simulink model "Bands8"  (R2018a)
settings: Solver=VariableStepAuto  StartTime=0.0  StopTime=0.007  RelTol=1e-3
undefined symbols (not defined in the file): fdesignblkfcn, G1, G2, G3, G4, G5, G6, G7, G8, gcbh, get, T
libraries: dspsrcs4 x1, dspxfrm3 x1, dspobslib x1
(part 1 of 3)
settings Model: Creator=Daniel  LastModifiedBy=Daniel

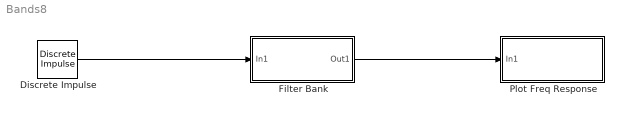
== system Bands8 ==
  Discrete Impulse : dspsrcs4/Discrete  Impulse  Delay=0  SampleTime=T  FrameSample=128  OutputFrames=off  dataType=double  isSigned=on  wordLen=16  udDataType=sfix(16)  fracBitsMode=Best precision  numFracBits=15  OutDataTypeStr=double  LastOutDataTypeStr=double
  "Filter Bank " : Subsystem
  Plot Freq Response : Subsystem
  wires:
  "Filter Bank "/1(Out1) -> Plot Freq Response/1(In1)
  Discrete Impulse/1 -> "Filter Bank "/1(In1)

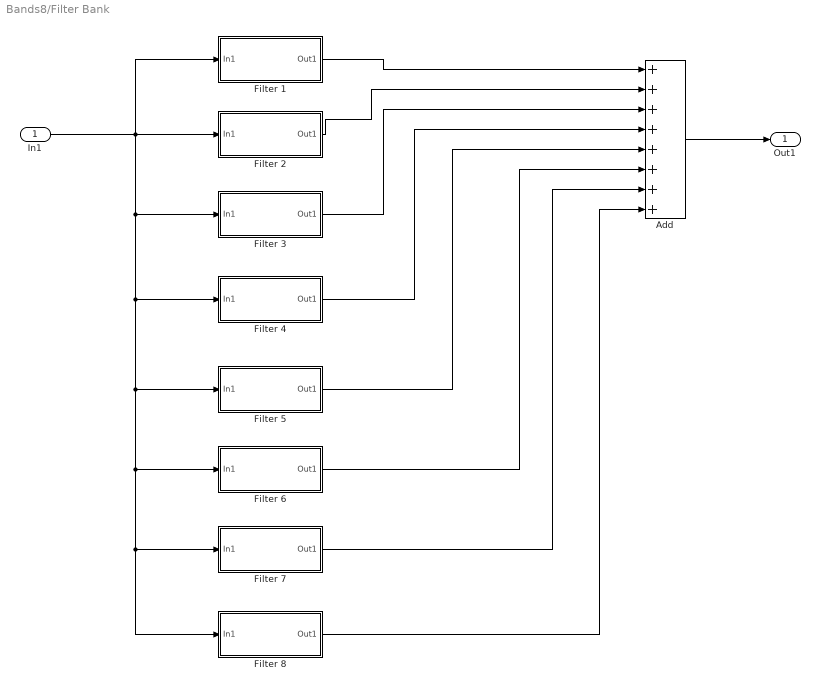
== system Bands8/Filter Bank  ==
  In1 : Inport
  Add : Sum  Inputs=++++++++
  Filter 1 : Subsystem
  Filter 2 : Subsystem
  Filter 3 : Subsystem
  Filter 4 : Subsystem
  Filter 5 : Subsystem
  Filter 6 : Subsystem
  Filter 7 : Subsystem
  Filter 8 : Subsystem
  Out1 : Outport
  wires:
  In1/1 -> Filter 3/1(In1), Filter 6/1(In1), Filter 8/1(In1), Filter 7/1(In1), Filter 5/1(In1), Filter 4/1(In1), Filter 1/1(In1), Filter 2/1(In1)
  Add/1 -> Out1/1
  Filter 1/1(Out1) -> Add/1
  Filter 2/1(Out1) -> Add/2
  Filter 3/1(Out1) -> Add/3
  Filter 4/1(Out1) -> Add/4
  Filter 5/1(Out1) -> Add/5
  Filter 6/1(Out1) -> Add/6
  Filter 7/1(Out1) -> Add/7
  Filter 8/1(Out1) -> Add/8

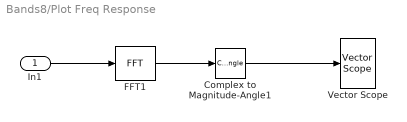
== system Bands8/Plot Freq Response ==
  In1 : Inport
  Complex to Magnitude-Angle1 : ComplexToMagnitudeAngle  Output=Magnitude
  FFT1 : dspxfrm3/FFT  FFTImplementation=Auto  CompMethod=Table lookup  TableOpt=NEW  TableOptActive=Speed  BitRevOrder=off  Normalize=off  InheritFFTLength=on  FFTLength=64  WrapInput=on  roundingMode=Floor  overflowMode=off  firstCoeffDataTypeStr=Inherit: Same word length as input  firstCoeffLastDataTypeStr=Inherit: Same word length as input  outputMin=[]  outputMax=[]
  Vector Scope : dspobslib/Vector Scope  ScopeProperties=off  Domain=Frequency  HorizSpan=1  DisplayProperties=off  AxisGrid=on  Memory=off  FrameNumber=off  AxisLegend=off  AxisZoom=off  OpenScopeAtSimStart=on  OpenScopeImmediately=off  FigPos=get(0,'defaultfigureposition')  AxisProperties=on  XUnits=Hertz  XRange=[0...Fs/2]  InheritXIncr=on  XIncr=1  XLabel=Samples  XLimit=Auto  XMin=0  XMax=1  XStart=0  YUnits=dB  YLabel=|Magnitude (dB)|  LineProperties=off  XAxisParamsVer=6.9
      settings: SourceProductName=DSP System Toolbox  SourceProductBaseCode=DS  YMin=0.0723692553519949  YMax=69.3188381671759
  wires:
  In1/1 -> FFT1/1
  FFT1/1 -> Complex to Magnitude-Angle1/1
  Complex to Magnitude-Angle1/1 -> Vector Scope/1

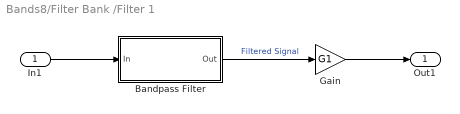
== system Bands8/Filter Bank /Filter 1 ==
  In1 : Inport
  Bandpass Filter : Subsystem  DialogController=fdesignblkfcn  InitFcn=fdesignblkfcn(gcbh, {'InitFcn'});  mask(Bandpass Filter){}
      mask help: Design a bandpass filter
      settings: CopyFcn=fdesignblkfcn(gcbh, {'CopyFcn'});
      mask Help: helpview(mapfilelocation('dsp'), 'dspbandpassfilter');
      mask Display: disp('Bandpass');
  Gain : Gain  Gain=G1
  Out1 : Outport
  wires:
  Bandpass Filter/1(Out) -> Gain/1  "Filtered Signal"
  In1/1 -> Bandpass Filter/1(In)
  Gain/1 -> Out1/1

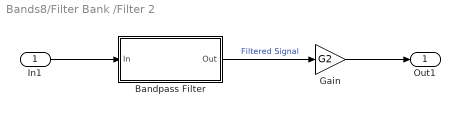
== system Bands8/Filter Bank /Filter 2 ==
  In1 : Inport
  Bandpass Filter : Subsystem  DialogController=fdesignblkfcn  InitFcn=fdesignblkfcn(gcbh, {'InitFcn'});  mask(Bandpass Filter){}
      mask help: Design a bandpass filter
      settings: CopyFcn=fdesignblkfcn(gcbh, {'CopyFcn'});
      mask Help: helpview(mapfilelocation('dsp'), 'dspbandpassfilter');
      mask Display: disp('Bandpass');
  Gain : Gain  Gain=G2
  Out1 : Outport
  wires:
  Bandpass Filter/1(Out) -> Gain/1  "Filtered Signal"
  In1/1 -> Bandpass Filter/1(In)
  Gain/1 -> Out1/1

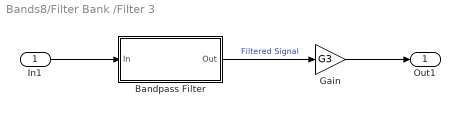
== system Bands8/Filter Bank /Filter 3 ==
  In1 : Inport
  Bandpass Filter : Subsystem  DialogController=fdesignblkfcn  InitFcn=fdesignblkfcn(gcbh, {'InitFcn'});  mask(Bandpass Filter){}
      mask help: Design a bandpass filter
      settings: CopyFcn=fdesignblkfcn(gcbh, {'CopyFcn'});
      mask Help: helpview(mapfilelocation('dsp'), 'dspbandpassfilter');
      mask Display: disp('Bandpass');
  Gain : Gain  Gain=G3
  Out1 : Outport
  wires:
  Bandpass Filter/1(Out) -> Gain/1  "Filtered Signal"
  In1/1 -> Bandpass Filter/1(In)
  Gain/1 -> Out1/1

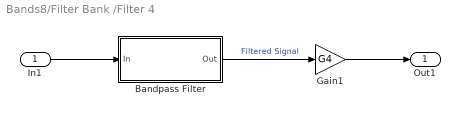
== system Bands8/Filter Bank /Filter 4 ==
  In1 : Inport
  Bandpass Filter : Subsystem  DialogController=fdesignblkfcn  InitFcn=fdesignblkfcn(gcbh, {'InitFcn'});  mask(Bandpass Filter){}
      mask help: Design a bandpass filter
      settings: CopyFcn=fdesignblkfcn(gcbh, {'CopyFcn'});
      mask Help: helpview(mapfilelocation('dsp'), 'dspbandpassfilter');
      mask Display: disp('Bandpass');
  Gain1 : Gain  Gain=G4
  Out1 : Outport
  wires:
  Bandpass Filter/1(Out) -> Gain1/1  "Filtered Signal"
  In1/1 -> Bandpass Filter/1(In)
  Gain1/1 -> Out1/1

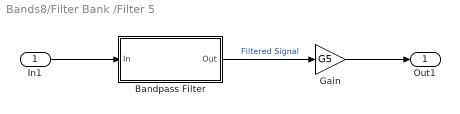
== system Bands8/Filter Bank /Filter 5 ==
  In1 : Inport
  Bandpass Filter : Subsystem  DialogController=fdesignblkfcn  InitFcn=fdesignblkfcn(gcbh, {'InitFcn'});  mask(Bandpass Filter){}
      mask help: Design a bandpass filter
      settings: CopyFcn=fdesignblkfcn(gcbh, {'CopyFcn'});
      mask Help: helpview(mapfilelocation('dsp'), 'dspbandpassfilter');
      mask Display: disp('Bandpass');
  Gain : Gain  Gain=G5
  Out1 : Outport
  wires:
  Bandpass Filter/1(Out) -> Gain/1  "Filtered Signal"
  In1/1 -> Bandpass Filter/1(In)
  Gain/1 -> Out1/1

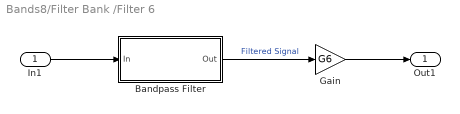
== system Bands8/Filter Bank /Filter 6 ==
  In1 : Inport
  Bandpass Filter : Subsystem  DialogController=fdesignblkfcn  InitFcn=fdesignblkfcn(gcbh, {'InitFcn'});  mask(Bandpass Filter){}
      mask help: Design a bandpass filter
      settings: CopyFcn=fdesignblkfcn(gcbh, {'CopyFcn'});
      mask Help: helpview(mapfilelocation('dsp'), 'dspbandpassfilter');
      mask Display: disp('Bandpass');
  Gain : Gain  Gain=G6
  Out1 : Outport
  wires:
  Bandpass Filter/1(Out) -> Gain/1  "Filtered Signal"
  In1/1 -> Bandpass Filter/1(In)
  Gain/1 -> Out1/1

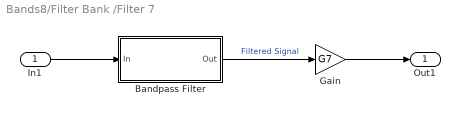
== system Bands8/Filter Bank /Filter 7 ==
  In1 : Inport
  Bandpass Filter : Subsystem  DialogController=fdesignblkfcn  InitFcn=fdesignblkfcn(gcbh, {'InitFcn'});  mask(Bandpass Filter){}
      mask help: Design a bandpass filter
      settings: CopyFcn=fdesignblkfcn(gcbh, {'CopyFcn'});
      mask Help: helpview(mapfilelocation('dsp'), 'dspbandpassfilter');
      mask Display: disp('Bandpass');
  Gain : Gain  Gain=G7
  Out1 : Outport
  wires:
  Bandpass Filter/1(Out) -> Gain/1  "Filtered Signal"
  In1/1 -> Bandpass Filter/1(In)
  Gain/1 -> Out1/1

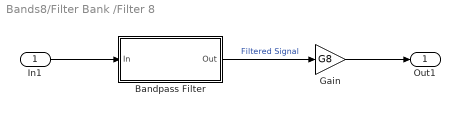
== system Bands8/Filter Bank /Filter 8 ==
  In1 : Inport
  Bandpass Filter : Subsystem  DialogController=fdesignblkfcn  InitFcn=fdesignblkfcn(gcbh, {'InitFcn'});  mask(Bandpass Filter){}
      mask help: Design a bandpass filter
      settings: CopyFcn=fdesignblkfcn(gcbh, {'CopyFcn'});
      mask Help: helpview(mapfilelocation('dsp'), 'dspbandpassfilter');
      mask Display: disp('Bandpass');
  Gain : Gain  Gain=G8
  Out1 : Outport
  wires:
  Bandpass Filter/1(Out) -> Gain/1  "Filtered Signal"
  In1/1 -> Bandpass Filter/1(In)
  Gain/1 -> Out1/1

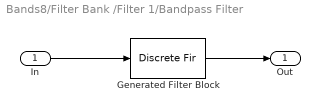
== system Bands8/Filter Bank /Filter 1/Bandpass Filter ==
  In : Inport
  Generated Filter Block : DiscreteFir  Tag=BlockMethodSubSystem  Coefficients=[-2.53930029891187237e-07 -1.39559102605358572e-06 -2.84299483017687342e-06 -5.63366029087786887e-06 -9.93418523252795173e-06 -1.63262241167292025e-05 -2.53229182196880342e-05 -3.74615020978339851e-05 -5.32173930372331465e-05 -7.29568465211660012e-05 -9.68737933684415595e-05 -0.000124931683125113687 -0.00015681338014041069 -0.000191885237263291733 -0.000229185274636913711 -0.000267438086672588211 -0.00030510213081918786 -0.000340448931074167395 -0.000371674915276808235 -0.000397035900377556484 -0.000414997858746321514 -0.000424390837332173617 -0.000424552406867539196 -0.000415441291437595474 -0.000397710773607891409 -0.000372726626144151538 -0.000342521253232423077 -0.000309679841562358091 -0.000277164576810850756 -0.000248082207234006594 -0.000225416218156756723 -0.000211744216275208176 -0.000208966862918188854 -0.000218076447132134477 -0.000238994846827390351 -0.000270497948353842961 -0.000310248957171879139 -0.000354942812809242456 -0.000400556891204730827 -0.00044269382199962719 -0.000476988183563495426 -0.000499537674052677808 -0.000507322673525113224 -0.000498561824487811912 -0.00047296866351605692 -0.000431870714973490999 -0.000378168748972630513 -0.000316131232422133337 -0.000251029791549493863 -0.000188645826868923355 -0.000134691640223129274 -9.41976040149720647e-05 -7.09370598389049377e-05 -6.69421117819960778e-05 -8.21813444080733409e-05 -0.000114432839276154899 -0.000159391227369712216 -0.00021100185817266243 -0.000262010585315348076 -0.000304675813254562291 -0.000331580963336122834 -0.000336461450709168151 -0.000314959039759978422 -0.000265213509228286637 -0.000188218441252340581 -8.78851377662456936e-05 2.92099411288585617e-05 0.000154386436678911681 0.000277687081250680974 0.000388896191038075561 0.000478646902205445658 0.000539501637954981983 0.000566882498331736009 0.000559739851257062631 0.000520868402043777462 0.000456814929229864923 0.00037736254208088697 0.000294625411855347914 0.000221830011900583555 0.000171902935068576315 0.000156009848128120879 0.000182207624058549342 0.0002543665133675509 0.000371498801018969415 0.000527592092942231507 0.000711995732851345353 0.000910346215381272741 0.00110596061419998906 0.00128156526883401595 0.0014211858626177994 0.00151199457068968693 0.00154590450599108959 0.00152071810325938922 0.00144067624870333581 0.00131631339020723908 0.00116359846846875409 0.00100241868471331961 0.000854544265290840344 0.000741273237086345431 0.000681007898100268383 0.000687030150247728471 0.000765738827078513715 0.000915571094494847934 0.00112676517528357634 0.00138203478965703429 0.00165812528110964672 0.00192812131304162396 0.00216428271439720677 0.00234111556354382137 0.00243834253748546718 0.00244343223745481335 0.00235337945449937656 0.00217549765889713583 0.00192708639446824729 0.00163395441061191878 0.00132791161748281421 0.0010434616699280851 0.000814032276633034095 0.000668146283307399563 0.000625965471708478296 0.000696614472810574677 0.000876627069478319414 0.00114974173512448919 0.00148813551384881617 0.00185502239612887971 0.0022083873073804371 0.00250548459341652348 0.00270762816029507161 0.00278474295050331819 0.00271915229050226706 0.00250813545339127145 0.00216491077514798262 0.00171785923810186718 0.00120799799622387351 0.000684909192349874674 0.000201516718921184221 -0.000191750037285460769 -0.000452770773023137814 -0.000552868026635460526 -0.000480646680445765643 -0.000244047619589907541 0.000129698376657387928 0.000596302676878664498 0.00109868251229961085 0.00157286112913479167 0.00195490915368107818 0.00218818529469917353 0.00223006952081876691 0.00205740277421887462 0.00166996080451258704 0.00109148191802953178 0.000368026141386225024 -0.000436264972918116143 -0.00124563987037357897 -0.00198080432235124473 -0.00256773857419659475 -0.00294629966950761026 -0.00307762328595569991 -0.00294943688007411877 -0.00257859024723299142 -0.00201039845224116427 -0.00131473241744564043 -0.000579160565752079629 0.000100210449749504773 0.000629257761509122724 ...(+7776 chars)]  InputProcessing=Columns as channels (frame based)
  Out : Outport
  wires:
  In/1 -> Generated Filter Block/1
  Generated Filter Block/1 -> Out/1

== system Bands8/Filter Bank /Filter 2/Bandpass Filter ==
  In : Inport
  Generated Filter Block : DiscreteFir  Tag=BlockMethodSubSystem  Coefficients=[5.30723377584483384e-07 1.19776025299245422e-07 -6.58666814243359492e-07 -2.10184937499317927e-06 -3.80071412837854187e-06 -4.77030737376980244e-06 -3.60752748263828817e-06 9.8377529791277464e-07 9.37008612682571497e-06 2.01366487998416324e-05 2.96399309223321596e-05 3.24168797364042378e-05 2.27076001482423253e-05 -3.06291617442429908e-06 -4.35133518348442195e-05 -9.03494749044171815e-05 -0.00012844376567534461 -0.000138797008783600657 -0.000104341873841668319 -1.73641334657300264e-05 0.000113796392106753987 0.000261644012740544951 0.000382460343799901519 0.000426175957788699526 0.000351754309323357693 0.00014414363060047885 -0.000172803095520407982 -0.000533141603176159515 -0.000839051655717063818 -0.000984304192496592966 -0.000886151695194846629 -0.000516813307086107709 7.60138140550270877e-05 0.000768601080925578354 0.00138457637020248823 0.0017389679864161648 0.00169221884114556607 0.00119850542377333293 0.000332219187134425115 -0.000718673327499120456 -0.00169441624530897021 -0.00233134178585766736 -0.00243742020123851244 -0.00195276910492362516 -0.000975171746587716608 0.000259791084594337713 0.00144064738834942746 0.00226698220028754812 0.00253550136911478638 0.00219837581578178308 0.00137496823527629244 0.000312588427325724105 -0.000691538286465870778 -0.00138195267532977028 -0.00162038054139924969 -0.00142029201054611419 -0.00092986712383753378 -0.000370391768836097785 4.74136635708194014e-05 0.000198998363661905095 8.64711633867901739e-05 -0.000170180625553737933 -0.000387152391434042063 -0.000395337512606723778 -0.000113203060701307377 0.000414187914448908032 0.0010256837693975293 0.0015010840945719698 0.00164383093519635329 0.00135818726051138662 0.000691136558506094743 -0.00017795765529278945 -0.00099731471041618531 -0.00153071220866774198 -0.0016407601022300519 -0.00133599592128368018 -0.000763695472209581332 -0.000150883456110647364 0.000283982434914520636 0.000414583473623001656 0.000252977366501809574 -5.98292005412435024e-05 -0.000315597168299764947 -0.000328699492852185284 -1.82968757413036072e-05 0.000550630331995880201 0.00118517161793123943 0.0016359087993694536 0.00169486539637159444 0.00128156480240376454 0.000482386695778048524 -0.000473984259822812781 -0.00129727193707246109 -0.00174219842880573694 -0.00169960712308197116 -0.00123593630199435702 -0.000564605610108467144 4.03132480643026453e-05 0.000354461383987730698 0.000293567948180090328 -5.30682883096933943e-05 -0.000460694601034692221 -0.000664794740545620612 -0.000476496925185968987 0.000129303915370603526 0.00099044232732715628 0.00181078474993610623 0.0022716359211521122 0.00215825340059078857 0.00145084268916968696 0.000342048188231852701 -0.000828609592228680709 -0.00169971398367218499 -0.0020240731940255525 -0.00176187421545964521 -0.00109266574939980354 -0.000339811677352434426 0.000163617530490524436 0.00021399897958842884 -0.000175612894430011377 -0.000777462718787295341 -0.00124203799996296387 -0.00124639640798968705 -0.000638308098113204493 0.000483738537630139947 0.00179047745844618657 0.00283793219080955353 0.00323634941169399348 0.00280558498218436755 0.00165366253702235147 0.000144232615041272846 -0.00123742873460524886 -0.00206885395150543114 -0.00215230658598597685 -0.00158837047993960561 -0.000729546641924390133 -3.03121248014422388e-05 0.000147073273093880524 -0.000308142066843700353 -0.00119799748596727653 -0.00208794955970169642 -0.00248311789622449692 -0.00203953203545851648 -0.00072421707723355753 0.00114432389636555105 0.00299724856337217974 0.00422303415514823071 0.00440175861443647867 0.00347237390406136479 0.00176335898487808233 -0.000129642359509899704 -0.0015739431743452062 -0.00214728773267066839 -0.00180262072572315063 -0.000881061329522545792 3.57740247822426439e-05 0.000377167609049017087 -0.000163060353712528398 -0.00147645251314596783 -0.00306005405948222729 -0.00420555726573881069 -0.0042863071883782319 -0.0030277776456050739 -0.000649252489836452118 0.00218727089689484296 0.00460861797830670362 ...(+7704 chars)]  InputProcessing=Columns as channels (frame based)
  Out : Outport
  wires:
  In/1 -> Generated Filter Block/1
  Generated Filter Block/1 -> Out/1

== system Bands8/Filter Bank /Filter 3/Bandpass Filter ==
  In : Inport
  Generated Filter Block : DiscreteFir  Tag=BlockMethodSubSystem  Coefficients=[-3.46201291617982891e-07 -5.86611112234273637e-07 -2.41741984152941371e-07 1.20791507789705158e-06 3.30494329138109444e-06 4.1512282543008902e-06 1.30140810431467984e-06 -5.82630993974713999e-06 -1.36044355713132795e-05 -1.46322733437421093e-05 -2.56550758661671922e-06 2.06690810150529475e-05 4.10923335268599581e-05 3.82848301264029759e-05 5.76304377198918899e-07 -5.91839307061305442e-05 -0.00010168544067447155 -8.20090873520503235e-05 1.41866403887614566e-05 0.000143903259263821506 0.000217038694213804245 0.000150829729796436149 -5.93206566654167259e-05 -0.000305337596749154303 -0.000410488581801839809 -0.000244389859351880746 0.000159213396989669608 0.000574912101890447049 0.000698473924532872696 0.0003540129613048671 -0.00033786305610963548 -0.000970447183460975186 -0.00107808046298802328 -0.000462037788693976496 0.000605376727589594394 0.00147635242700873632 0.00151413158768721177 0.000544746185621797154 -0.000941486599442781279 -0.00202556144268727133 -0.00193191111895547451 -0.000578878895913442944 0.00128362272030344417 0.00249415532167592945 0.00222264397141814238 0.000549956429480658059 -0.00152915515841818388 -0.00271949315025976721 -0.00226661221026338818 -0.000459186431730172219 0.00155889618626674654 0.00254621718854197449 0.00197264412728214529 0.000325546765602279886 -0.00128090736355890148 -0.00189207662484576272 -0.00132396965552946744 -0.000181114244285260437 0.000682140649406868908 0.000811227743875355713 0.000412552699099926498 6.05022858028783571e-05 0.000134464894590950626 0.000476303317643663566 0.00055837264585203441 1.1776020603567606e-05 -0.000951787080700099868 -0.00161665587918511777 -0.00131701745167209791 -3.06145282859419986e-05 0.00149324602067355287 0.00222374713286032288 0.00160815717957572737 1.17113455929636789e-05 -0.00152278289427042364 -0.00202731027324335334 -0.00129676154937243622 1.62541500288403479e-05 0.000956973267075066341 0.00101354690523491669 0.0004494769600238468 -2.56165556241975574e-05 6.06740093436498659e-05 0.000509197779912389198 0.000649113595665043105 3.47062192513899184e-06 -0.00116968038240433322 -0.00197151451713661018 -0.00157064413771034308 4.17155257112663449e-05 0.00190498439001578288 0.00273604598663523737 0.00189717899995100504 -8.44642683637651122e-05 -0.00188434020676971764 -0.00236550389000231287 -0.00140452498739484241 9.60954525619534282e-05 0.000999246099305423552 0.000857470504231963733 0.000196895221767656069 -6.13386269951409071e-05 0.000481515161670153841 0.00127268441651979137 0.00128065015464159547 -1.09823474924118077e-05 -0.00196521622846692603 -0.00313382575323793624 -0.00238448129049292391 8.95511896926997773e-05 0.0027535683496484626 0.00380643842099204167 0.00253514459682385685 -0.000134786868683011151 -0.00235492864097556131 -0.00277161557499916097 -0.00150092583567564713 0.000119243612355649189 0.000757819057602526877 0.00023177210978141561 -0.000428724489594280059 -4.37622997584607076e-05 0.00147508133509223114 0.00285338154869280028 0.00248495445211128476 -5.97673722887831946e-05 -0.00337336326949724992 -0.00508889097323463394 -0.00369883357934726754 0.000141847492727349304 0.00395458147333596285 0.00523778041501598429 0.00333004412016764872 -0.000159402965056991191 -0.00269958946436277486 -0.00284948868692788682 -0.00126703056614365099 9.86322471379051386e-05 -0.00010934887579805544 -0.00137471090913409777 -0.00180001691947203777 1.54766219233574371e-05 0.00337776150188023871 0.00570592704805264646 0.00456023929342399322 -0.000129041650654218343 -0.00558099650178511125 -0.00803305985605905909 -0.0055975040034679565 0.00018488481027514509 0.00542602328879135745 0.00681532306703067428 0.00405615360824676269 -0.000151584142725344229 -0.00252499914509178624 -0.00194161228756274608 -0.00016725168888930949 4.10847120265476958e-05 -0.00224007698319337104 -0.00493082995781331593 -0.00464138448917522824 9.49810922370646565e-05 0.00689115880488391872 0.0108154714283432204 0.00818225582028434852 -0.000189566448013943958 -0.00908206340820759232 ...(+6053 chars)]  InputProcessing=Columns as channels (frame based)
  Out : Outport
  wires:
  In/1 -> Generated Filter Block/1
  Generated Filter Block/1 -> Out/1
